simulink model "sim_tase_2025_att_ctrl"  (R2020a)
settings: Solver=ode4  StartTime=0.0  StopTime=30.0  FixedStep=0.01  RelTol=1e-3
values from neighbouring files (symbols this model uses):
  alfa_i_init = zeros(3, NF)    [init_tase_2025_att_ctrl.m]
  beta_ij_init = zeros(3, NF)    [init_tase_2025_att_ctrl.m]
  c1 = 2.5    [init_tase_2025_att_ctrl.m]
  c1_diff_sigma_bar_w = diag([12; 12; 12])    [init_tase_2025_att_ctrl.m]
  c1_diff_ui = diag([25; 30; 20])    [init_tase_2025_att_ctrl.m]
  c2 = 2.0    (= 2)    [init_tase_2025_att_ctrl.m]
  c2_diff_sigma_bar_w = diag([12; 12; 12])    [init_tase_2025_att_ctrl.m]
  c2_diff_ui = diag([50; 50; 10])    [init_tase_2025_att_ctrl.m]
  c3_diff_sigma_bar_w = diag([15; 15; 15])    [init_tase_2025_att_ctrl.m]
  c3_diff_ui = diag([15; 15; 10])    [init_tase_2025_att_ctrl.m]
  dw_aa_t = 0.2 * ones(3, 5) + ( 1.0 - 0.2 ) * rand(3, 5)    [init_tase_2025_att_ctrl.m]
  dw_ff_t = [ 0.4 * ones(1, 5) + ( 1.0 - 0.4 ) * rand(1, 5);                      0.4 * ones(1, 5) + ( 1.0 - 0.4 ) * rand(1, 5);                      0.2 * ones(1, 5) + ( 0.6 - 0.2 ) * rand(1, 5) ]    [init_tase_2025_att_ctrl.m]
  dw_phi_t = ( - pi / 2 ) * ones(3, 5) + ( pi / 2 - ( - pi / 2 ) ) * rand(3, 5)    [init_tase_2025_att_ctrl.m]
  dwci_init = zeros(3,5)    [init_tase_2025_att_ctrl.m]
  err_wi_init = zeros(3, NF)    [init_tase_2025_att_ctrl.m]
  eta_1_ij_init = zeros(3, NF)    [init_tase_2025_att_ctrl.m]
  eta_2_ij_init = zeros(3, NF)    [init_tase_2025_att_ctrl.m]
  h1w = diag([20.0; 20.0; 20.0])    [init_tase_2025_att_ctrl.m]
  h2w = diag([30.0; 35.0; 35.0])    [init_tase_2025_att_ctrl.m]
  h3w = diag([30.0; 25.0; 30.0])    [init_tase_2025_att_ctrl.m]
  Ji = zeros(3,3,NF)    [init_tase_2025_att_ctrl.m]
  k_1_ij_hat_init = zeros(3, NF)    [init_tase_2025_att_ctrl.m]
  k_1_ij_init = zeros(3, NF)    [init_tase_2025_att_ctrl.m]
  k_1_ij_lower = zeros(3, NF)    [init_tase_2025_att_ctrl.m]
  k_1_ij_upper = zeros(3, NF)    [init_tase_2025_att_ctrl.m]
  k_2_ij_init = zeros(3, NF)    [init_tase_2025_att_ctrl.m]
  k_2_ij_lower = zeros(3, NF)    [init_tase_2025_att_ctrl.m]
  k_2_ij_upper = zeros(3, NF)    [init_tase_2025_att_ctrl.m]
  Lamd_diff_sigma_bar_w = 0.8    [init_tase_2025_att_ctrl.m]
  Lamd_diff_ui = 0.8    [init_tase_2025_att_ctrl.m]
  mu1 = 0.2    [init_tase_2025_att_ctrl.m]
  mu2 = 0.2    [init_tase_2025_att_ctrl.m]
  mu_d_w = 100    [init_tase_2025_att_ctrl.m]
  phi_ij_init = ones(3, NF)    [init_tase_2025_att_ctrl.m]
  pos0 = zeros(3, 1)    [init_tase_2025_att_ctrl.m]
  PZ0 = P0(3)    [init_tase_2025_att_ctrl.m]
  PZ1 = 10    [init_tase_2025_att_ctrl.m]
  q_ij_hat_init = zeros(3, NF)    [init_tase_2025_att_ctrl.m]
  Qci_init = repmat([1;0;0;0],1,NF)    [init_tase_2025_att_ctrl.m]
  R0 = 4    [init_tase_2025_att_ctrl.m]
  R1 = 8    [init_tase_2025_att_ctrl.m]
  Rci_init = zeros(3,3,NF)    [init_tase_2025_att_ctrl.m]
  Ri_init = zeros(3,3,NF)    [init_tase_2025_att_ctrl.m]
  Rx2 = 10    [init_tase_2025_att_ctrl.m]
  Ry2 = 6    [init_tase_2025_att_ctrl.m]
  Rz2 = 4    [init_tase_2025_att_ctrl.m]
  T0 = 0    [init_tase_2025_att_ctrl.m]
  T1 = tseq1    (= 10)    [init_tase_2025_att_ctrl.m]
  T2 = tseq1 + tseq12 + tseq2    (= 30)    [init_tase_2025_att_ctrl.m]
  T_ij = repmat([60.0; 60.0; 60.0], 1, NF)    [init_tase_2025_att_ctrl.m]
  ui_init = zeros(3,NF)    [init_tase_2025_att_ctrl.m]
  vel0 = zeros(3, 1)    [init_tase_2025_att_ctrl.m]
  wci_init = zeros(3,5)    [init_tase_2025_att_ctrl.m]
  zeta_diff_sigma_bar_w = 0.3    [init_tase_2025_att_ctrl.m]
  zeta_diff_ui = 0.05    [init_tase_2025_att_ctrl.m]
undefined symbols (not defined in the file or in its folder): cal_frac_squ, p_alfaw1, p_alfaw2, q_alfaw1, q_alfaw2, Qei_init, Qi_init, Rei_init, V_Phi_Rei_init, wei_init, wi_init
(part 4 of 5)

== matlab function sim_tase_2025_att_ctrl/combine wei Qei Rei ==
  data: wei_1 input; wei_vec output; wei_2 input; wei_3 input; wei_4 input; wei_5 input; Qei_1 input; Qei_2 input; Qei_3 input; Qei_4 input; Qei_5 input; Rei_1 input; Rei_2 input; Rei_3 input; Rei_4 input; Rei_5 input; Qei_vec output; Rei_vec output
function [wei_vec, Qei_vec, Rei_vec] = fcn(wei_1, wei_2, wei_3, wei_4, wei_5, ...
                                                                            Qei_1, Qei_2, Qei_3, Qei_4, Qei_5, ...
                                                                            Rei_1, Rei_2, Rei_3, Rei_4, Rei_5)
%%%% 合并姿态角速率误差/四元数误差/姿态旋转矩阵误差
wei_vec = zeros(3,5);
wei_vec(:,1) = wei_1(:);
wei_vec(:,2) = wei_2(:);
wei_vec(:,3) = wei_3(:);
wei_vec(:,4) = wei_4(:);
wei_vec(:,5) = wei_5(:);

Qei_vec = zeros(4,5);
Qei_vec(:,1) = Qei_1(:);
Qei_vec(:,2) = Qei_2(:);
Qei_vec(:,3) = Qei_3(:);
Qei_vec(:,4) = Qei_4(:);
Qei_vec(:,5) = Qei_5(:);

Rei_vec = zeros(3,3,5);
Rei_vec(:,:,1) = Rei_1;
Rei_vec(:,:,2) = Rei_2;
Rei_vec(:,:,3) = Rei_3;
Rei_vec(:,:,4) = Rei_4;
Rei_vec(:,:,5) = Rei_5;

== matlab function sim_tase_2025_att_ctrl/cal Ri agent 1 ==
  data: Ri_1 output; Qi_vec input
function Ri_1 = fcn(Qi_vec)
%%%% 使用罗德里格公式由四元数Qi求解Ri
iiuav = 1;
thetai_tmp = Qi_vec(1,iiuav);
qi_tmp = Qi_vec(2:4,iiuav);
Ri_1 = ((thetai_tmp^2) - (qi_tmp')*qi_tmp) * eye(3,3) ...
            + 2 * qi_tmp * (qi_tmp') ...
            - 2 * thetai_tmp * cal_askew_mat(qi_tmp);

end

== matlab function sim_tase_2025_att_ctrl/cal Ri agent 2 ==
  data: Ri_2 output; Qi_vec input
function Ri_2 = fcn(Qi_vec)
%%%% 使用罗德里格公式由四元数Qi求解Ri
iiuav = 2;
thetai_tmp = Qi_vec(1,iiuav);
qi_tmp = Qi_vec(2:4,iiuav);
Ri_2 = ((thetai_tmp^2) - (qi_tmp')*qi_tmp) * eye(3,3) ...
            + 2 * qi_tmp * (qi_tmp') ...
            - 2 * thetai_tmp * cal_askew_mat(qi_tmp);

end

== matlab function sim_tase_2025_att_ctrl/combine phi_ij ==
  data: phi_ij_1 input; phi_ij_vec output; phi_ij_2 input; phi_ij_3 input; phi_ij_4 input; phi_ij_5 input
function phi_ij_vec = fcn(phi_ij_1, phi_ij_2, phi_ij_3, phi_ij_4, phi_ij_5)
%%%% 合并性能调节函数
phi_ij_vec = [phi_ij_1(:), phi_ij_2(:), phi_ij_3(:), phi_ij_4(:), phi_ij_5(:)];

== matlab function sim_tase_2025_att_ctrl/cal Ri agent 3 ==
  data: Ri_3 output; Qi_vec input
function Ri_3 = fcn(Qi_vec)
%%%% 使用罗德里格公式由四元数Qi求解Ri
iiuav = 3;
thetai_tmp = Qi_vec(1,iiuav);
qi_tmp = Qi_vec(2:4,iiuav);
Ri_3 = ((thetai_tmp^2) - (qi_tmp')*qi_tmp) * eye(3,3) ...
            + 2 * qi_tmp * (qi_tmp') ...
            - 2 * thetai_tmp * cal_askew_mat(qi_tmp);

end

== matlab function sim_tase_2025_att_ctrl/cal Ri agent 4 ==
  data: Ri_4 output; Qi_vec input
function Ri_4 = fcn(Qi_vec)
%%%% 使用罗德里格公式由四元数Qi求解Ri
iiuav = 4;
thetai_tmp = Qi_vec(1,iiuav);
qi_tmp = Qi_vec(2:4,iiuav);
Ri_4 = ((thetai_tmp^2) - (qi_tmp')*qi_tmp) * eye(3,3) ...
            + 2 * qi_tmp * (qi_tmp') ...
            - 2 * thetai_tmp * cal_askew_mat(qi_tmp);

end

== matlab function sim_tase_2025_att_ctrl/cal Ri agent 5 ==
  data: Ri_5 output; Qi_vec input
function Ri_5 = fcn(Qi_vec)
%%%% 使用罗德里格公式由四元数Qi求解Ri
iiuav = 5;
thetai_tmp = Qi_vec(1,iiuav);
qi_tmp = Qi_vec(2:4,iiuav);
Ri_5 = ((thetai_tmp^2) - (qi_tmp')*qi_tmp) * eye(3,3) ...
            + 2 * qi_tmp * (qi_tmp') ...
            - 2 * thetai_tmp * cal_askew_mat(qi_tmp);

end

== matlab function sim_tase_2025_att_ctrl/cal Qci agent 1 ==
  data: Qi_vec input; Qci_1 output; Qei_vec input
function Qci_1 = fcn(Qi_vec, Qei_vec)
%%%% 更新期望指令四元数
iiuav = 1;

sigma1 = Qi_vec(1,iiuav);
q1 = Qi_vec(2:4,iiuav);
sigma2 = Qei_vec(1,iiuav);
q2 = -Qei_vec(2:4,iiuav);

sigma = sigma1*sigma2 - (q1')*q2;
q = sigma1*q2 + sigma2*q1 + cal_askew_mat(q1)*q2;
Qci_1 = [sigma; q];

end

== matlab function sim_tase_2025_att_ctrl/cal Rci agent 1 ==
  data: Rci_1 output; Qci input
function Rci_1 = fcn(Qci)
%%%% 使用罗德里格公式由四元数Qci求解Rci
thetaci_tmp = Qci(1,1);
qci_tmp = Qci(2:4,1);
Rci_1 = ((thetaci_tmp^2) - (qci_tmp')*qci_tmp) * eye(3,3) ...
                + 2 * qci_tmp * (qci_tmp') ...
                - 2 * thetaci_tmp * cal_askew_mat(qci_tmp);

end

== matlab function sim_tase_2025_att_ctrl/cal Qci agent 2 ==
  data: Qi_vec input; Qci_2 output; Qei_vec input
function Qci_2 = fcn(Qi_vec, Qei_vec)
%%%% 更新期望指令四元数
iiuav = 2;
sigma1 = Qi_vec(1,iiuav);
q1 = Qi_vec(2:4,iiuav);
sigma2 = Qei_vec(1,iiuav);
q2 = -Qei_vec(2:4,iiuav);

sigma = sigma1*sigma2 - (q1')*q2;
q = sigma1*q2 + sigma2*q1 + cal_askew_mat(q1)*q2;
Qci_2 = [sigma; q];

end

== matlab function sim_tase_2025_att_ctrl/cal Rci agent 2 ==
  data: Rci_2 output; Qci input
function Rci_2 = fcn(Qci)
%%%% 使用罗德里格公式由四元数Qci求解Rci

thetaci_tmp = Qci(1,1);
qci_tmp = Qci(2:4,1);
Rci_2 = ((thetaci_tmp^2) - (qci_tmp')*qci_tmp) * eye(3,3) ...
                + 2 * qci_tmp * (qci_tmp') ...
                - 2 * thetaci_tmp * cal_askew_mat(qci_tmp);

end

== matlab function sim_tase_2025_att_ctrl/cal Qci agent 3 ==
  data: Qi_vec input; Qci_3 output; Qei_vec input
function Qci_3 = fcn(Qi_vec, Qei_vec)
%%%% 更新期望指令四元数
iiuav = 3;
sigma1 = Qi_vec(1,iiuav);
q1 = Qi_vec(2:4,iiuav);
sigma2 = Qei_vec(1,iiuav);
q2 = -Qei_vec(2:4,iiuav);

sigma = sigma1*sigma2 - (q1')*q2;
q = sigma1*q2 + sigma2*q1 + cal_askew_mat(q1)*q2;
Qci_3 = [sigma; q];

end

== matlab function sim_tase_2025_att_ctrl/cal Rci agent 3 ==
  data: Rci_3 output; Qci input
function Rci_3 = fcn(Qci)
%%%% 使用罗德里格公式由四元数Qci求解Rci
thetaci_tmp = Qci(1,1);
qci_tmp = Qci(2:4,1);
Rci_3 = ((thetaci_tmp^2) - (qci_tmp')*qci_tmp) * eye(3,3) ...
                + 2 * qci_tmp * (qci_tmp') ...
                - 2 * thetaci_tmp * cal_askew_mat(qci_tmp);

end

== matlab function sim_tase_2025_att_ctrl/cal Qci agent 4 ==
  data: Qi_vec input; Qci_4 output; Qei_vec input
function Qci_4 = fcn(Qi_vec, Qei_vec)
%%%% 更新期望指令四元数
iiuav = 4;
sigma1 = Qi_vec(1,iiuav);
q1 = Qi_vec(2:4,iiuav);
sigma2 = Qei_vec(1,iiuav);
q2 = -Qei_vec(2:4,iiuav);

sigma = sigma1*sigma2 - (q1')*q2;
q = sigma1*q2 + sigma2*q1 + cal_askew_mat(q1)*q2;
Qci_4 = [sigma; q];

end

== matlab function sim_tase_2025_att_ctrl/cal Rci agent 4 ==
  data: Rci_4 output; Qci input
function Rci_4 = fcn(Qci)
%%%% 使用罗德里格公式由四元数Qci求解Rci
thetaci_tmp = Qci(1,1);
qci_tmp = Qci(2:4,1);
Rci_4 = ((thetaci_tmp^2) - (qci_tmp')*qci_tmp) * eye(3,3) ...
                + 2 * qci_tmp * (qci_tmp') ...
                - 2 * thetaci_tmp * cal_askew_mat(qci_tmp);

end

== matlab function sim_tase_2025_att_ctrl/cal Qci agent 5 ==
  data: Qi_vec input; Qci_5 output; Qei_vec input
function Qci_5 = fcn(Qi_vec, Qei_vec)
%%%% 更新期望指令四元数
iiuav = 5;
sigma1 = Qi_vec(1,iiuav);
q1 = Qi_vec(2:4,iiuav);
sigma2 = Qei_vec(1,iiuav);
q2 = -Qei_vec(2:4,iiuav);

sigma = sigma1*sigma2 - (q1')*q2;
q = sigma1*q2 + sigma2*q1 + cal_askew_mat(q1)*q2;
Qci_5 = [sigma; q];

end

== matlab function sim_tase_2025_att_ctrl/cal Rci agent 5 ==
  data: Rci_5 output; Qci_vec input
function Rci_5 = fcn(Qci_vec)
%%%% 使用罗德里格公式由四元数Qci求解Rci
thetaci_tmp = Qci_vec(1,1);
qci_tmp = Qci_vec(2:4,1);
Rci_5 = ((thetaci_tmp^2) - (qci_tmp')*qci_tmp) * eye(3,3) ...
                + 2 * qci_tmp * (qci_tmp') ...
                - 2 * thetaci_tmp * cal_askew_mat(qci_tmp);

end

== matlab function sim_tase_2025_att_ctrl/combine Qci Rci ==
  data: Qci_1 input; Qci_vec output; Qci_2 input; Qci_3 input; Qci_4 input; Qci_5 input; Rci_1 input; Rci_2 input; Rci_3 input; Rci_4 input; Rci_5 input; Rci_vec output
function [Qci_vec, Rci_vec] = fcn(Qci_1, Qci_2, Qci_3, Qci_4, Qci_5, ...
                                                            Rci_1, Rci_2, Rci_3, Rci_4, Rci_5)
%%%% 合并四元数和姿态旋转矩阵
Qci_vec = zeros(4,5);
Qci_vec(:,1) = Qci_1(:);
Qci_vec(:,2) = Qci_2(:);
Qci_vec(:,3) = Qci_3(:);
Qci_vec(:,4) = Qci_4(:);
Qci_vec(:,5) = Qci_5(:);

Rci_vec = zeros(3,3,5);
Rci_vec(:,:,1) = Rci_1;
Rci_vec(:,:,2) = Rci_2;
Rci_vec(:,:,3) = Rci_3;
Rci_vec(:,:,4) = Rci_4;
Rci_vec(:,:,5) = Rci_5;

== matlab function sim_tase_2025_att_ctrl/cal k_1_ij agent 1 ==
  data: mu1 input; k_1_ij_lower input; k_1_ij_node_1 output; k_1_ij_upper input; phi_ij_vec input; tsim input
function k_1_ij_node_1 = fcn(mu1, k_1_ij_lower, k_1_ij_upper, phi_ij_vec, tsim)
%%%% 计算预设性能函数
iiuav = 1;
k_1_ij_node_1 = zeros(3,1);
for jj = 1:3
    k_1_ij_node_1(jj) = k_1_ij_lower(jj, iiuav) + ( k_1_ij_upper(jj, iiuav) - k_1_ij_lower(jj, iiuav) ) * phi_ij_vec(jj, iiuav);
%     k_1_ij_node_1(jj) = k_1_ij_lower(jj, iiuav) + ( k_1_ij_upper(jj, iiuav) - k_1_ij_lower(jj, iiuav) ) * phi_ij_vec(jj, iiuav) * exp( - mu1 * tsim );
%     k_1_ij_node_1(jj) = k_1_ij_lower(jj, iiuav) + ( k_1_ij_upper(jj, iiuav) - k_1_ij_lower(jj, iiuav) ) * exp( - mu1 * tsim );
end

== matlab function sim_tase_2025_att_ctrl/depart eta_1_ij 5 ==
  data: y output; x input
function y = fcn(x)
y = x(:,5);

end

== matlab function sim_tase_2025_att_ctrl/depart eta_1_ij 1 ==
  data: y output; x input
function y = fcn(x)
y = x(:,1);

end

== matlab function sim_tase_2025_att_ctrl/depart eta_1_ij 2 ==
  data: y output; x input
function y = fcn(x)
y = x(:,2);

end

== matlab function sim_tase_2025_att_ctrl/depart eta_1_ij 3 ==
  data: y output; x input
function y = fcn(x)
y = x(:,3);

end

== matlab function sim_tase_2025_att_ctrl/depart eta_1_ij 4 ==
  data: y output; x input
function y = fcn(x)
y = x(:,4);

end

== matlab function sim_tase_2025_att_ctrl/depart eta_2_ij 5 ==
  data: y output; x input
function y = fcn(x)
y = x(:,5);

end

== matlab function sim_tase_2025_att_ctrl/depart eta_2_ij 1 ==
  data: y output; x input
function y = fcn(x)
y = x(:,1);

end

== matlab function sim_tase_2025_att_ctrl/depart eta_2_ij 2 ==
  data: y output; x input
function y = fcn(x)
y = x(:,2);

end

== matlab function sim_tase_2025_att_ctrl/depart eta_2_ij 3 ==
  data: y output; x input
function y = fcn(x)
y = x(:,3);

end

== matlab function sim_tase_2025_att_ctrl/depart eta_2_ij 4 ==
  data: y output; x input
function y = fcn(x)
y = x(:,4);

end

== matlab function sim_tase_2025_att_ctrl/cal V_Phi_Rei agent 1 ==
  data: Rei_vec input; V_Phi_Rei_1 output
function V_Phi_Rei_1 = fcn(Rei_vec)
%%%% 更新姿态旋转指数坐标
iiuav = 1;
phiei = 0.5 * ( trace( Rei_vec(:,:,iiuav) ) - 1 );
V_Phi_Rei_1 = ( phiei / ( 2 * sin( phiei ) ) ) * ...
                            cal_back_askew_mat( Rei_vec(:,:,iiuav) - ( Rei_vec(:,:,iiuav)' ) );
end

== matlab function sim_tase_2025_att_ctrl/cal V_Phi_Rei agent 2 ==
  data: Rei_vec input; V_Phi_Rei_2 output
function V_Phi_Rei_2 = fcn(Rei_vec)
%%%% 更新姿态旋转指数坐标
iiuav = 2;
phiei = 0.5 * ( trace( Rei_vec(:,:,iiuav) ) - 1 );
V_Phi_Rei_2 = ( phiei / ( 2 * sin( phiei ) ) ) * ...
                            cal_back_askew_mat( Rei_vec(:,:,iiuav) - ( Rei_vec(:,:,iiuav)' ) );
end

== matlab function sim_tase_2025_att_ctrl/cal V_Phi_Rei agent 3 ==
  data: Rei_vec input; V_Phi_Rei_3 output
function V_Phi_Rei_3 = fcn(Rei_vec)
%%%% 更新姿态旋转指数坐标
iiuav = 3;
phiei = 0.5 * ( trace( Rei_vec(:,:,iiuav) ) - 1 );
V_Phi_Rei_3 = ( phiei / ( 2 * sin( phiei ) ) ) * ...
                            cal_back_askew_mat( Rei_vec(:,:,iiuav) - ( Rei_vec(:,:,iiuav)' ) );
end

== matlab function sim_tase_2025_att_ctrl/cal V_Phi_Rei agent 4 ==
  data: Rei_vec input; V_Phi_Rei_4 output
function V_Phi_Rei_4 = fcn(Rei_vec)
%%%% 更新姿态旋转指数坐标
iiuav = 4;
phiei = 0.5 * ( trace( Rei_vec(:,:,iiuav) ) - 1 );
V_Phi_Rei_4 = ( phiei / ( 2 * sin( phiei ) ) ) * ...
                            cal_back_askew_mat( Rei_vec(:,:,iiuav) - ( Rei_vec(:,:,iiuav)' ) );
end

== matlab function sim_tase_2025_att_ctrl/cal V_Phi_Rei agent 5 ==
  data: Rei_vec input; V_Phi_Rei_5 output
function V_Phi_Rei_5 = fcn(Rei_vec)
%%%% 更新姿态旋转指数坐标
iiuav = 5;
phiei = 0.5 * ( trace( Rei_vec(:,:,iiuav) ) - 1 );
V_Phi_Rei_5 = ( phiei / ( 2 * sin( phiei ) ) ) * ...
                            cal_back_askew_mat( Rei_vec(:,:,iiuav) - ( Rei_vec(:,:,iiuav)' ) );
end

== matlab function sim_tase_2025_att_ctrl/cal k_1_ij agent 2 ==
  data: mu1 input; k_1_ij_lower input; k_1_ij_node_2 output; k_1_ij_upper input; phi_ij_vec input; tsim input
function k_1_ij_node_2 = fcn(mu1, k_1_ij_lower, k_1_ij_upper, phi_ij_vec, tsim)
%%%% 计算预设性能函数
iiuav = 2;
k_1_ij_node_2 = zeros(3,1);
for jj = 1:3
    k_1_ij_node_2(jj) = k_1_ij_lower(jj, iiuav) + ( k_1_ij_upper(jj, iiuav) - k_1_ij_lower(jj, iiuav) ) * phi_ij_vec(jj, iiuav);
%     k_1_ij_node_2(jj) = k_1_ij_lower(jj, iiuav) + ( k_1_ij_upper(jj, iiuav) - k_1_ij_lower(jj, iiuav) ) * phi_ij_vec(jj, iiuav) * exp( - mu1 * tsim );
%     k_1_ij_node_2(jj) = k_1_ij_lower(jj, iiuav) + ( k_1_ij_upper(jj, iiuav) - k_1_ij_lower(jj, iiuav) ) * exp( - mu1 * tsim );
end

== matlab function sim_tase_2025_att_ctrl/cal differentiator d_sigma_bar_w_hat agent 3/choose sigma_bar_w ==
  data: x input; y output
function y = fcn(x)
iiuav = 3;
y = x(:,iiuav);

== matlab function sim_tase_2025_att_ctrl/cal differentiator d_sigma_bar_w_hat agent 3/trans to column20 ==
  data: x input; y output
function y = fcn(x)
y = x(:);

== matlab function sim_tase_2025_att_ctrl/cal differentiator d_sigma_bar_w_hat agent 3/trans to column21 ==
  data: x input; y output
function y = fcn(x)
y = x(:);

== matlab function sim_tase_2025_att_ctrl/cal differentiator d_sigma_bar_w_hat agent 3/trans to column22 ==
  data: x input; y output
function y = fcn(x)
y = x(:);

== matlab function sim_tase_2025_att_ctrl/cal differentiator d_sigma_bar_w_hat agent 3/trans to column23 ==
  data: x input; y output
function y = fcn(x)
y = x(:);

== matlab function sim_tase_2025_att_ctrl/combine Qci Rci1 ==
  data: V_Phi_Rei_1 input; V_Phi_Rei_vec output; V_Phi_Rei_2 input; V_Phi_Rei_3 input; V_Phi_Rei_4 input; V_Phi_Rei_5 input
function V_Phi_Rei_vec = fcn(V_Phi_Rei_1, V_Phi_Rei_2, V_Phi_Rei_3, V_Phi_Rei_4, V_Phi_Rei_5)
%%%% 合并LogSO3空间的辅助姿态误差向量
V_Phi_Rei_vec = [V_Phi_Rei_1(:), V_Phi_Rei_2(:), V_Phi_Rei_3(:), V_Phi_Rei_4(:), V_Phi_Rei_5(:)];

== matlab function sim_tase_2025_att_ctrl/depart Qe1 ==
  data: y output; x input
function y = fcn(x)
y = x(:,1);

end

== matlab function sim_tase_2025_att_ctrl/depart Qe2 ==
  data: y output; x input
function y = fcn(x)
y = x(:,2);

end

== matlab function sim_tase_2025_att_ctrl/depart Qe3 ==
  data: y output; x input
function y = fcn(x)
y = x(:,3);

end

== matlab function sim_tase_2025_att_ctrl/depart Qe4 ==
  data: y output; x input
function y = fcn(x)
y = x(:,4);

end

== matlab function sim_tase_2025_att_ctrl/depart Qe5 ==
  data: y output; x input
function y = fcn(x)
y = x(:,5);

end

== matlab function sim_tase_2025_att_ctrl/depart we1 ==
  data: y output; x input
function y = fcn(x)
y = x(:,1);

end

== matlab function sim_tase_2025_att_ctrl/depart we2 ==
  data: y output; x input
function y = fcn(x)
y = x(:,2);

end

== matlab function sim_tase_2025_att_ctrl/depart we3 ==
  data: y output; x input
function y = fcn(x)
y = x(:,3);

end

== matlab function sim_tase_2025_att_ctrl/depart we4 ==
  data: y output; x input
function y = fcn(x)
y = x(:,4);

end

== matlab function sim_tase_2025_att_ctrl/cal k_1_ij agent 3 ==
  data: mu1 input; k_1_ij_lower input; k_1_ij_node_3 output; k_1_ij_upper input; phi_ij_vec input; tsim input
function k_1_ij_node_3 = fcn(mu1, k_1_ij_lower, k_1_ij_upper, phi_ij_vec, tsim)
%%%% 计算预设性能函数
iiuav = 3;
k_1_ij_node_3 = zeros(3,1);
for jj = 1:3
    k_1_ij_node_3(jj) = k_1_ij_lower(jj, iiuav) + ( k_1_ij_upper(jj, iiuav) - k_1_ij_lower(jj, iiuav) ) * phi_ij_vec(jj, iiuav);
%     k_1_ij_node_3(jj) = k_1_ij_lower(jj, iiuav) + ( k_1_ij_upper(jj, iiuav) - k_1_ij_lower(jj, iiuav) ) * phi_ij_vec(jj, iiuav) * exp( - mu1 * tsim );
%     k_1_ij_node_3(jj) = k_1_ij_lower(jj, iiuav) + ( k_1_ij_upper(jj, iiuav) - k_1_ij_lower(jj, iiuav) ) * exp( - mu1 * tsim );
end

== matlab function sim_tase_2025_att_ctrl/depart we5 ==
  data: y output; x input
function y = fcn(x)
y = x(:,5);

end

== matlab function sim_tase_2025_att_ctrl/depart V_Phi_Re5 ==
  data: y output; x input
function y = fcn(x)
y = x(:,5);

end

== matlab function sim_tase_2025_att_ctrl/depart V_Phi_Re1 ==
  data: y output; x input
function y = fcn(x)
y = x(:,1);

end

== matlab function sim_tase_2025_att_ctrl/depart V_Phi_Re2 ==
  data: y output; x input
function y = fcn(x)
y = x(:,2);

end

== matlab function sim_tase_2025_att_ctrl/depart V_Phi_Re3 ==
  data: y output; x input
function y = fcn(x)
y = x(:,3);

end

== matlab function sim_tase_2025_att_ctrl/depart V_Phi_Re4 ==
  data: y output; x input
function y = fcn(x)
y = x(:,4);

end

== matlab function sim_tase_2025_att_ctrl/cal differentiator d_sigma_bar_w_hat agent 3/trans to column24 ==
  data: x input; y output
function y = fcn(x)
y = x(:);

== matlab function sim_tase_2025_att_ctrl/cal differentiator d_sigma_bar_w_hat agent 3/trans to column25 ==
  data: x input; y output
function y = fcn(x)
y = x(:);

== matlab function sim_tase_2025_att_ctrl/cal differentiator d_sigma_bar_w_hat agent 4/cal differentiator ==
  data: c1 input; d_sigma_bar_v_hat output; d_dsigma_bar_v_hat output; d_d2sigma_bar_v_hat output; c2 input; c3 input; chi_t input; sigma_bar_v_sig_1 input; sigma_bar_v_sig_2 input; sigma_bar_v_sig_3 input; sigma_bar_v_sig_4 input; sigma_bar_v_sig_5 input; sigma_bar_v_sig_6 input; d_sigma_bar_v_hat input; d2_sigma_bar_v_hat input
function [d_sigma_bar_v_hat, d_dsigma_bar_v_hat, d_d2sigma_bar_v_hat] = fcn(c1, c2, c3, chi_t, sigma_bar_v_sig_1, sigma_bar_v_sig_2, sigma_bar_v_sig_3, ...
                                                                                                                                                sigma_bar_v_sig_4, sigma_bar_v_sig_5, sigma_bar_v_sig_6, d_sigma_bar_v_hat, d2_sigma_bar_v_hat)
d_d2sigma_bar_v_hat = -chi_t .* c1 * sigma_bar_v_sig_1(:) - (1 - chi_t) .* c1 * sigma_bar_v_sig_2(:);
d_dsigma_bar_v_hat = -chi_t .* c2 * sigma_bar_v_sig_3(:) - (1 - chi_t) .* c2 * sigma_bar_v_sig_4(:) + d2_sigma_bar_v_hat(:);
d_sigma_bar_v_hat = -chi_t .* c3 * sigma_bar_v_sig_5(:) - (1 - chi_t) .* c3 * sigma_bar_v_sig_6(:) + d_sigma_bar_v_hat(:);

== matlab function sim_tase_2025_att_ctrl/cal differentiator d_sigma_bar_w_hat agent 4/cal sig ==
  data: x input; z output; y input
function z = fcn(x, y)
z = x(:) .* sign(y(:));

== matlab function sim_tase_2025_att_ctrl/cal differentiator d_sigma_bar_w_hat agent 4/cal sig1 ==
  data: x input; z output; y input
function z = fcn(x, y)
z = x(:) .* sign(y(:));

== matlab function sim_tase_2025_att_ctrl/cal differentiator d_sigma_bar_w_hat agent 4/cal sig2 ==
  data: x input; z output; y input
function z = fcn(x, y)
z = x(:) .* sign(y(:));

== matlab function sim_tase_2025_att_ctrl/cal differentiator d_sigma_bar_w_hat agent 4/cal sig3 ==
  data: x input; z output; y input
function z = fcn(x, y)
z = x(:) .* sign(y(:));

== matlab function sim_tase_2025_att_ctrl/cal k_1_ij agent 4 ==
  data: mu1 input; k_1_ij_lower input; k_1_ij_node_4 output; k_1_ij_upper input; phi_ij_vec input; tsim input
function k_1_ij_node_4 = fcn(mu1, k_1_ij_lower, k_1_ij_upper, phi_ij_vec, tsim)
%%%% 计算预设性能函数
iiuav = 4;
k_1_ij_node_4 = zeros(3,1);
for jj = 1:3
    k_1_ij_node_4(jj) = k_1_ij_lower(jj, iiuav) + ( k_1_ij_upper(jj, iiuav) - k_1_ij_lower(jj, iiuav) ) * phi_ij_vec(jj, iiuav);
%     k_1_ij_node_4(jj) = k_1_ij_lower(jj, iiuav) + ( k_1_ij_upper(jj, iiuav) - k_1_ij_lower(jj, iiuav) ) * phi_ij_vec(jj, iiuav) * exp( - mu1 * tsim );
%     k_1_ij_node_4(jj) = k_1_ij_lower(jj, iiuav) + ( k_1_ij_upper(jj, iiuav) - k_1_ij_lower(jj, iiuav) ) * exp( - mu1 * tsim );
end

== matlab function sim_tase_2025_att_ctrl/cal differentiator d_sigma_bar_w_hat agent 4/cal sig4 ==
  data: x input; z output; y input
function z = fcn(x, y)
z = x(:) .* sign(y(:));

== matlab function sim_tase_2025_att_ctrl/cal differentiator d_sigma_bar_w_hat agent 4/cal sig5 ==
  data: x input; z output; y input
function z = fcn(x, y)
z = x(:) .* sign(y(:));

== matlab function sim_tase_2025_att_ctrl/cal differentiator d_sigma_bar_w_hat agent 4/choose sigma_bar_w ==
  data: x input; y output
function y = fcn(x)
iiuav = 4;
y = x(:,iiuav);

== matlab function sim_tase_2025_att_ctrl/cal differentiator d_sigma_bar_w_hat agent 4/trans to column20 ==
  data: x input; y output
function y = fcn(x)
y = x(:);

== matlab function sim_tase_2025_att_ctrl/cal differentiator d_sigma_bar_w_hat agent 4/trans to column21 ==
  data: x input; y output
function y = fcn(x)
y = x(:);

== matlab function sim_tase_2025_att_ctrl/cal differentiator d_sigma_bar_w_hat agent 4/trans to column22 ==
  data: x input; y output
function y = fcn(x)
y = x(:);

== matlab function sim_tase_2025_att_ctrl/cal differentiator d_sigma_bar_w_hat agent 4/trans to column23 ==
  data: x input; y output
function y = fcn(x)
y = x(:);

== matlab function sim_tase_2025_att_ctrl/cal differentiator d_sigma_bar_w_hat agent 4/trans to column24 ==
  data: x input; y output
function y = fcn(x)
y = x(:);

== matlab function sim_tase_2025_att_ctrl/cal differentiator d_sigma_bar_w_hat agent 4/trans to column25 ==
  data: x input; y output
function y = fcn(x)
y = x(:);

== matlab function sim_tase_2025_att_ctrl/cal differentiator d_sigma_bar_w_hat agent 5/cal differentiator ==
  data: c1 input; d_sigma_bar_v_hat output; d_dsigma_bar_v_hat output; d_d2sigma_bar_v_hat output; c2 input; c3 input; chi_t input; sigma_bar_v_sig_1 input; sigma_bar_v_sig_2 input; sigma_bar_v_sig_3 input; sigma_bar_v_sig_4 input; sigma_bar_v_sig_5 input; sigma_bar_v_sig_6 input; d_sigma_bar_v_hat input; d2_sigma_bar_v_hat input
function [d_sigma_bar_v_hat, d_dsigma_bar_v_hat, d_d2sigma_bar_v_hat] = fcn(c1, c2, c3, chi_t, sigma_bar_v_sig_1, sigma_bar_v_sig_2, sigma_bar_v_sig_3, ...
                                                                                                                                                sigma_bar_v_sig_4, sigma_bar_v_sig_5, sigma_bar_v_sig_6, d_sigma_bar_v_hat, d2_sigma_bar_v_hat)
d_d2sigma_bar_v_hat = -chi_t .* c1 * sigma_bar_v_sig_1(:) - (1 - chi_t) .* c1 * sigma_bar_v_sig_2(:);
d_dsigma_bar_v_hat = -chi_t .* c2 * sigma_bar_v_sig_3(:) - (1 - chi_t) .* c2 * sigma_bar_v_sig_4(:) + d2_sigma_bar_v_hat(:);
d_sigma_bar_v_hat = -chi_t .* c3 * sigma_bar_v_sig_5(:) - (1 - chi_t) .* c3 * sigma_bar_v_sig_6(:) + d_sigma_bar_v_hat(:);

== matlab function sim_tase_2025_att_ctrl/cal differentiator d_sigma_bar_w_hat agent 5/cal sig ==
  data: x input; z output; y input
function z = fcn(x, y)
z = x(:) .* sign(y(:));

== matlab function sim_tase_2025_att_ctrl/cal differentiator d_sigma_bar_w_hat agent 5/cal sig1 ==
  data: x input; z output; y input
function z = fcn(x, y)
z = x(:) .* sign(y(:));

== matlab function sim_tase_2025_att_ctrl/cal differentiator d_sigma_bar_w_hat agent 5/cal sig2 ==
  data: x input; z output; y input
function z = fcn(x, y)
z = x(:) .* sign(y(:));

== matlab function sim_tase_2025_att_ctrl/cal differentiator d_sigma_bar_w_hat agent 5/cal sig3 ==
  data: x input; z output; y input
function z = fcn(x, y)
z = x(:) .* sign(y(:));

== matlab function sim_tase_2025_att_ctrl/cal k_1_ij agent 5 ==
  data: mu1 input; k_1_ij_lower input; k_1_ij_node_5 output; k_1_ij_upper input; phi_ij_vec input; tsim input
function k_1_ij_node_5 = fcn(mu1, k_1_ij_lower, k_1_ij_upper, phi_ij_vec, tsim)
%%%% 计算预设性能函数
iiuav = 5;
k_1_ij_node_5 = zeros(3,1);
for jj = 1:3
    k_1_ij_node_5(jj) = k_1_ij_lower(jj, iiuav) + ( k_1_ij_upper(jj, iiuav) - k_1_ij_lower(jj, iiuav) ) * phi_ij_vec(jj, iiuav);
%     k_1_ij_node_5(jj) = k_1_ij_lower(jj, iiuav) + ( k_1_ij_upper(jj, iiuav) - k_1_ij_lower(jj, iiuav) ) * phi_ij_vec(jj, iiuav) * exp( - mu1 * tsim );
%     k_1_ij_node_5(jj) = k_1_ij_lower(jj, iiuav) + ( k_1_ij_upper(jj, iiuav) - k_1_ij_lower(jj, iiuav) ) * exp( - mu1 * tsim );
end

== matlab function sim_tase_2025_att_ctrl/cal differentiator d_sigma_bar_w_hat agent 5/cal sig4 ==
  data: x input; z output; y input
function z = fcn(x, y)
z = x(:) .* sign(y(:));

== matlab function sim_tase_2025_att_ctrl/cal differentiator d_sigma_bar_w_hat agent 5/cal sig5 ==
  data: x input; z output; y input
function z = fcn(x, y)
z = x(:) .* sign(y(:));

== matlab function sim_tase_2025_att_ctrl/cal differentiator d_sigma_bar_w_hat agent 5/choose sigma_bar_w ==
  data: x input; y output
function y = fcn(x)
iiuav = 5;
y = x(:,iiuav);

== matlab function sim_tase_2025_att_ctrl/cal differentiator d_sigma_bar_w_hat agent 5/trans to column20 ==
  data: x input; y output
function y = fcn(x)
y = x(:);

== matlab function sim_tase_2025_att_ctrl/cal differentiator d_sigma_bar_w_hat agent 5/trans to column21 ==
  data: x input; y output
function y = fcn(x)
y = x(:);

== matlab function sim_tase_2025_att_ctrl/cal differentiator d_sigma_bar_w_hat agent 5/trans to column22 ==
  data: x input; y output
function y = fcn(x)
y = x(:);

== matlab function sim_tase_2025_att_ctrl/cal differentiator d_sigma_bar_w_hat agent 5/trans to column23 ==
  data: x input; y output
function y = fcn(x)
y = x(:);

== matlab function sim_tase_2025_att_ctrl/cal differentiator d_sigma_bar_w_hat agent 5/trans to column24 ==
  data: x input; y output
function y = fcn(x)
y = x(:);

== matlab function sim_tase_2025_att_ctrl/cal differentiator d_sigma_bar_w_hat agent 5/trans to column25 ==
  data: x input; y output
function y = fcn(x)
y = x(:);

== matlab function sim_tase_2025_att_ctrl/cal dw_hat agent 1 ==
  data: h3w input; Ji input; d_sigma_bar_w_vec input; sigma_bar_w_hat_vec input; dw_hat_1 output
function dw_hat_1 = fcn(h3w, Ji, d_sigma_bar_w_vec, sigma_bar_w_hat_vec)
%%%% 计算扰动观测值dw_hat
iiuav = 1;
dw_hat_1 = Ji(:,:,iiuav) * d_sigma_bar_w_vec(:,iiuav) + h3w * sigma_bar_w_hat_vec(:,iiuav);

== matlab function sim_tase_2025_att_ctrl/cal dw_hat agent 2 ==
  data: h3w input; Ji input; d_sigma_bar_w_vec input; sigma_bar_w_hat_vec input; dw_hat_2 output
function dw_hat_2 = fcn(h3w, Ji, d_sigma_bar_w_vec, sigma_bar_w_hat_vec)
%%%% 计算扰动观测值dw_hat
iiuav = 2;
dw_hat_2 = Ji(:,:,iiuav) * d_sigma_bar_w_vec(:,iiuav) + h3w * sigma_bar_w_hat_vec(:,iiuav);

== matlab function sim_tase_2025_att_ctrl/cal dw_hat agent 3 ==
  data: h3w input; Ji input; d_sigma_bar_w_vec input; sigma_bar_w_hat_vec input; dw_hat_3 output
function dw_hat_3 = fcn(h3w, Ji, d_sigma_bar_w_vec, sigma_bar_w_hat_vec)
%%%% 计算扰动观测值dw_hat
iiuav = 3;
dw_hat_3 = Ji(:,:,iiuav) * d_sigma_bar_w_vec(:,iiuav) + h3w * sigma_bar_w_hat_vec(:,iiuav);

== matlab function sim_tase_2025_att_ctrl/cal dw_hat agent 4 ==
  data: h3w input; Ji input; d_sigma_bar_w_vec input; sigma_bar_w_hat_vec input; dw_hat_4 output
function dw_hat_4 = fcn(h3w, Ji, d_sigma_bar_w_vec, sigma_bar_w_hat_vec)
%%%% 计算扰动观测值dw_hat
iiuav = 4;
dw_hat_4 = Ji(:,:,iiuav) * d_sigma_bar_w_vec(:,iiuav) + h3w * sigma_bar_w_hat_vec(:,iiuav);

== matlab function sim_tase_2025_att_ctrl/combine k_1_ij ==
  data: k_1_ij_node_1 input; k_1_ij_vec output; k_1_ij_node_2 input; k_1_ij_node_3 input; k_1_ij_node_4 input; k_1_ij_node_5 input
function k_1_ij_vec = fcn(k_1_ij_node_1, k_1_ij_node_2, k_1_ij_node_3, k_1_ij_node_4, k_1_ij_node_5)
%%%% 合并预设性能函数
k_1_ij_vec = [k_1_ij_node_1(:), k_1_ij_node_2(:), k_1_ij_node_3(:), k_1_ij_node_4(:), k_1_ij_node_5(:)];

== matlab function sim_tase_2025_att_ctrl/cal dw_hat agent 5 ==
  data: h3w input; Ji input; d_sigma_bar_w_vec input; sigma_bar_w_hat_vec input; dw_hat_5 output
function dw_hat_5 = fcn(h3w, Ji, d_sigma_bar_w_vec, sigma_bar_w_hat_vec)
%%%% 计算扰动观测值dw_hat
iiuav = 5;
dw_hat_5 = Ji(:,:,iiuav) * d_sigma_bar_w_vec(:,iiuav) + h3w * sigma_bar_w_hat_vec(:,iiuav);

== matlab function sim_tase_2025_att_ctrl/cal error dw_tilt ==
  data: dw_vec input; dw_hat_vec input; dw_tilt_vec output
function dw_tilt_vec = fcn(dw_vec, dw_hat_vec)
%%%% 计算扰动观测误差dw_tilt
dw_tilt_vec = zeros(3,5);
for iiuav = 1:5
    dw_tilt_vec(:,iiuav) = dw_vec(:,iiuav) - dw_hat_vec(:,iiuav);
end

== matlab function sim_tase_2025_att_ctrl/cal sigma_bar_w_hat agent 1 ==
  data: h1w input; h2w input; theta_sigma_bar_w_tilt_1_vec input; d_sigma_bar_w_hat_1 output; theta_sigma_bar_w_tilt_2_vec input; d_sigma_bar_w_vec input
function d_sigma_bar_w_hat_1 = fcn(h1w, h2w, theta_sigma_bar_w_tilt_1_vec, theta_sigma_bar_w_tilt_2_vec, d_sigma_bar_w_vec)
%%%% 计算扰动观测器中虚拟速度控制量观测值sigma_w_hat的微分方程
iiuav = 1;
d_sigma_bar_w_hat_1 = d_sigma_bar_w_vec(:,iiuav) + ...
                                            h1w * theta_sigma_bar_w_tilt_1_vec(:,iiuav) + ...
                                            h2w * theta_sigma_bar_w_tilt_2_vec(:,iiuav);

== matlab function sim_tase_2025_att_ctrl/cal sigma_bar_w_hat agent 2 ==
  data: h1w input; h2w input; theta_sigma_bar_w_tilt_1_vec input; d_sigma_bar_w_hat_2 output; theta_sigma_bar_w_tilt_2_vec input; d_sigma_bar_w_vec input
function d_sigma_bar_w_hat_2 = fcn(h1w, h2w, theta_sigma_bar_w_tilt_1_vec, theta_sigma_bar_w_tilt_2_vec, d_sigma_bar_w_vec)
%%%% 计算扰动观测器中虚拟速度控制量观测值sigma_v_hat的微分方程
iiuav = 2;
d_sigma_bar_w_hat_2 = d_sigma_bar_w_vec(:,iiuav) + ...
                                            h1w * theta_sigma_bar_w_tilt_1_vec(:,iiuav) + ...
                                            h2w * theta_sigma_bar_w_tilt_2_vec(:,iiuav);

== matlab function sim_tase_2025_att_ctrl/cal sigma_bar_w_hat agent 3 ==
  data: h1w input; h2w input; theta_sigma_bar_w_tilt_1_vec input; d_sigma_bar_w_hat_3 output; theta_sigma_bar_w_tilt_2_vec input; d_sigma_bar_w_vec input
function d_sigma_bar_w_hat_3 = fcn(h1w, h2w, theta_sigma_bar_w_tilt_1_vec, theta_sigma_bar_w_tilt_2_vec, d_sigma_bar_w_vec)
%%%% 计算扰动观测器中虚拟速度控制量观测值sigma_w_hat的微分方程
iiuav = 3;
d_sigma_bar_w_hat_3 = d_sigma_bar_w_vec(:,iiuav) + ...
                                            h1w * theta_sigma_bar_w_tilt_1_vec(:,iiuav) + ...
                                            h2w * theta_sigma_bar_w_tilt_2_vec(:,iiuav);

== matlab function sim_tase_2025_att_ctrl/cal sigma_bar_w_hat agent 4 ==
  data: h1w input; h2w input; theta_sigma_bar_w_tilt_1_vec input; d_sigma_bar_w_hat_4 output; theta_sigma_bar_w_tilt_2_vec input; d_sigma_bar_w_vec input
function d_sigma_bar_w_hat_4 = fcn(h1w, h2w, theta_sigma_bar_w_tilt_1_vec, theta_sigma_bar_w_tilt_2_vec, d_sigma_bar_w_vec)
%%%% 计算扰动观测器中虚拟速度控制量观测值sigma_w_hat的微分方程
iiuav = 4;
d_sigma_bar_w_hat_4 = d_sigma_bar_w_vec(:,iiuav) + ...
                                            h1w * theta_sigma_bar_w_tilt_1_vec(:,iiuav) + ...
                                            h2w * theta_sigma_bar_w_tilt_2_vec(:,iiuav);

== matlab function sim_tase_2025_att_ctrl/cal sigma_bar_w_hat agent 5 ==
  data: h1w input; h2w input; theta_sigma_bar_w_tilt_1_vec input; d_sigma_bar_w_hat_5 output; theta_sigma_bar_w_tilt_2_vec input; d_sigma_bar_w_vec input
function d_sigma_bar_w_hat_5 = fcn(h1w, h2w, theta_sigma_bar_w_tilt_1_vec, theta_sigma_bar_w_tilt_2_vec, d_sigma_bar_w_vec)
%%%% 计算扰动观测器中虚拟速度控制量观测值sigma_w_hat的微分方程
iiuav = 5;
d_sigma_bar_w_hat_5 = d_sigma_bar_w_vec(:,iiuav) + ...
                                            h1w * theta_sigma_bar_w_tilt_1_vec(:,iiuav) + ...
                                            h2w * theta_sigma_bar_w_tilt_2_vec(:,iiuav);

== matlab function sim_tase_2025_att_ctrl/cal sigma_w_bar ==
  data: sigma_bar_w_vec output; wi_vec input; sigma_w_vec input
function sigma_bar_w_vec = fcn(wi_vec, sigma_w_vec)
%%%% 计算姿态角速率跟踪误差
sigma_bar_w_vec = zeros(3,5);
for iiuav = 1:5
    sigma_bar_w_vec(:,iiuav) = wi_vec(:,iiuav) - sigma_w_vec(:,iiuav);
end

== matlab function sim_tase_2025_att_ctrl/cal theta_sigma_bar_w_tilt agent 1 ==
  data: alfa_theta_obs_w input; sigma_bar_w_tilt_squ_1_1 input; theta_sigma_bar_w_tilt_1_1 output; sigma_bar_w_tilt_squ_2_1 input; sigma_bar_w_tilt_vec input; theta_sigma_bar_w_tilt_2_1 output
function [theta_sigma_bar_w_tilt_1_1, theta_sigma_bar_w_tilt_2_1] = fcn(alfa_theta_obs_w, sigma_bar_w_tilt_squ_1_1, sigma_bar_w_tilt_squ_2_1, sigma_bar_w_tilt_vec)
%%%% 计算平滑递增函数
iiuav = 1;
theta_sigma_bar_w_tilt_1_1 = sigma_bar_w_tilt_squ_1_1(:) .* ( -1 + 2 ./ ( 1 + exp( -alfa_theta_obs_w .* sigma_bar_w_tilt_vec(:,iiuav) ) ) );
theta_sigma_bar_w_tilt_2_1 = sigma_bar_w_tilt_squ_2_1(:) .* ( -1 + 2 ./ ( 1 + exp( -alfa_theta_obs_w .* sigma_bar_w_tilt_vec(:,iiuav) ) ) );

== matlab function sim_tase_2025_att_ctrl/cal theta_sigma_bar_w_tilt agent 2 ==
  data: alfa_theta_obs_w input; sigma_bar_w_tilt_squ_1_2 input; theta_sigma_bar_w_tilt_1_2 output; sigma_bar_w_tilt_squ_2_2 input; sigma_bar_w_tilt_vec input; theta_sigma_bar_w_tilt_2_2 output
function [theta_sigma_bar_w_tilt_1_2, theta_sigma_bar_w_tilt_2_2] = fcn(alfa_theta_obs_w, sigma_bar_w_tilt_squ_1_2, sigma_bar_w_tilt_squ_2_2, sigma_bar_w_tilt_vec)
%%%% 计算平滑递增函数
iiuav = 2;
theta_sigma_bar_w_tilt_1_2 = sigma_bar_w_tilt_squ_1_2(:) .* ( -1 + 2 ./ ( 1 + exp( -alfa_theta_obs_w .* sigma_bar_w_tilt_vec(:,iiuav) ) ) );
theta_sigma_bar_w_tilt_2_2 = sigma_bar_w_tilt_squ_2_2(:) .* ( -1 + 2 ./ ( 1 + exp( -alfa_theta_obs_w .* sigma_bar_w_tilt_vec(:,iiuav) ) ) );

== matlab function sim_tase_2025_att_ctrl/cal theta_sigma_bar_w_tilt agent 3 ==
  data: alfa_theta_obs_w input; sigma_bar_w_tilt_squ_1_3 input; theta_sigma_bar_w_tilt_1_3 output; sigma_bar_w_tilt_squ_2_3 input; sigma_bar_w_tilt_vec input; theta_sigma_bar_w_tilt_2_3 output
function [theta_sigma_bar_w_tilt_1_3, theta_sigma_bar_w_tilt_2_3] = fcn(alfa_theta_obs_w, sigma_bar_w_tilt_squ_1_3, sigma_bar_w_tilt_squ_2_3, sigma_bar_w_tilt_vec)
%%%% 计算平滑递增函数
iiuav = 3;
theta_sigma_bar_w_tilt_1_3 = sigma_bar_w_tilt_squ_1_3(:) .* ( -1 + 2 ./ ( 1 + exp( -alfa_theta_obs_w .* sigma_bar_w_tilt_vec(:,iiuav) ) ) );
theta_sigma_bar_w_tilt_2_3 = sigma_bar_w_tilt_squ_2_3(:) .* ( -1 + 2 ./ ( 1 + exp( -alfa_theta_obs_w .* sigma_bar_w_tilt_vec(:,iiuav) ) ) );

== matlab function sim_tase_2025_att_ctrl/cal k_1_ij_hat agent 1 ==
  data: k_1_ij_lower input; k_1_ij_hat_node_1 output; k_1_ij_vec input
function k_1_ij_hat_node_1 = fcn(k_1_ij_lower, k_1_ij_vec)
%%%% 计算障碍函数
iiuav = 1;
k_1_ij_hat_node_1 = zeros(3,1);
for jj = 1:3
    k_1_ij_hat_node_1(jj) = (1/2) * ( k_1_ij_vec(jj,iiuav) + k_1_ij_lower(jj,iiuav) );
end

== matlab function sim_tase_2025_att_ctrl/cal theta_sigma_bar_w_tilt agent 4 ==
  data: alfa_theta_obs_w input; sigma_bar_w_tilt_squ_1_4 input; theta_sigma_bar_w_tilt_1_4 output; sigma_bar_w_tilt_squ_2_4 input; sigma_bar_w_tilt_vec input; theta_sigma_bar_w_tilt_2_4 output
function [theta_sigma_bar_w_tilt_1_4, theta_sigma_bar_w_tilt_2_4] = fcn(alfa_theta_obs_w, sigma_bar_w_tilt_squ_1_4, sigma_bar_w_tilt_squ_2_4, sigma_bar_w_tilt_vec)
%%%% 计算平滑递增函数
iiuav = 4;
theta_sigma_bar_w_tilt_1_4 = sigma_bar_w_tilt_squ_1_4(:) .* ( -1 + 2 ./ ( 1 + exp( -alfa_theta_obs_w .* sigma_bar_w_tilt_vec(:,iiuav) ) ) );
theta_sigma_bar_w_tilt_2_4 = sigma_bar_w_tilt_squ_2_4(:) .* ( -1 + 2 ./ ( 1 + exp( -alfa_theta_obs_w .* sigma_bar_w_tilt_vec(:,iiuav) ) ) );

== matlab function sim_tase_2025_att_ctrl/cal theta_sigma_bar_w_tilt agent 5 ==
  data: alfa_theta_obs_w input; sigma_bar_w_tilt_squ_1_5 input; theta_sigma_bar_w_tilt_1_5 output; sigma_bar_w_tilt_squ_2_5 input; sigma_bar_w_tilt_vec input; theta_sigma_bar_w_tilt_2_5 output
function [theta_sigma_bar_w_tilt_1_5, theta_sigma_bar_w_tilt_2_5] = fcn(alfa_theta_obs_w, sigma_bar_w_tilt_squ_1_5, sigma_bar_w_tilt_squ_2_5, sigma_bar_w_tilt_vec)
%%%% 计算平滑递增函数
iiuav = 5;
theta_sigma_bar_w_tilt_1_5 = sigma_bar_w_tilt_squ_1_5(:) .* ( -1 + 2 ./ ( 1 + exp( -alfa_theta_obs_w .* sigma_bar_w_tilt_vec(:,iiuav) ) ) );
theta_sigma_bar_w_tilt_2_5 = sigma_bar_w_tilt_squ_2_5(:) .* ( -1 + 2 ./ ( 1 + exp( -alfa_theta_obs_w .* sigma_bar_w_tilt_vec(:,iiuav) ) ) );

== matlab function sim_tase_2025_att_ctrl/choose ksi_est_err 11 ==
  data: x input; y output
function y = fcn(x)
iiuav = 1;
y = x(:,iiuav);

== matlab function sim_tase_2025_att_ctrl/choose ksi_est_err 12 ==
  data: x input; y output
function y = fcn(x)
iiuav = 1;
y = x(:,iiuav);

== matlab function sim_tase_2025_att_ctrl/choose ksi_est_err 13 ==
  data: x input; y output
function y = fcn(x)
iiuav = 2;
y = x(:,iiuav);

== matlab function sim_tase_2025_att_ctrl/choose ksi_est_err 14 ==
  data: x input; y output
function y = fcn(x)
iiuav = 2;
y = x(:,iiuav);

== matlab function sim_tase_2025_att_ctrl/choose ksi_est_err 15 ==
  data: x input; y output
function y = fcn(x)
iiuav = 3;
y = x(:,iiuav);

== matlab function sim_tase_2025_att_ctrl/choose ksi_est_err 16 ==
  data: x input; y output
function y = fcn(x)
iiuav = 3;
y = x(:,iiuav);

== matlab function sim_tase_2025_att_ctrl/choose ksi_est_err 17 ==
  data: x input; y output
function y = fcn(x)
iiuav = 4;
y = x(:,iiuav);

== matlab function sim_tase_2025_att_ctrl/choose ksi_est_err 18 ==
  data: x input; y output
function y = fcn(x)
iiuav = 4;
y = x(:,iiuav);

== matlab function sim_tase_2025_att_ctrl/cal k_1_ij_hat agent 2 ==
  data: k_1_ij_lower input; k_1_ij_hat_node_2 output; k_1_ij_vec input
function k_1_ij_hat_node_2 = fcn(k_1_ij_lower, k_1_ij_vec)
%%%% 计算障碍函数
iiuav = 2;
k_1_ij_hat_node_2 = zeros(3,1);
for jj = 1:3
    k_1_ij_hat_node_2(jj) = (1/2) * ( k_1_ij_vec(jj,iiuav) + k_1_ij_lower(jj,iiuav) );
end

== matlab function sim_tase_2025_att_ctrl/choose ksi_est_err 19 ==
  data: x input; y output
function y = fcn(x)
iiuav = 5;
y = x(:,iiuav);

== matlab function sim_tase_2025_att_ctrl/choose ksi_est_err 20 ==
  data: x input; y output
function y = fcn(x)
iiuav = 5;
y = x(:,iiuav);

== matlab function sim_tase_2025_att_ctrl/combine d_sigma_bar_v_est ==
  data: d_sigma_bar_w_est_1 input; d_sigma_bar_w_est_2 input; d_sigma_bar_w_est_3 input; d_sigma_bar_w_est_4 input; d_sigma_bar_w_est_5 input; d_sigma_bar_w_vec output
function d_sigma_bar_w_vec  = fcn(d_sigma_bar_w_est_1, d_sigma_bar_w_est_2, d_sigma_bar_w_est_3, d_sigma_bar_w_est_4, d_sigma_bar_w_est_5)
%%%% 合并用微分器求得的虚拟速度控制量导数
d_sigma_bar_w_vec = [d_sigma_bar_w_est_1(:), d_sigma_bar_w_est_2(:), d_sigma_bar_w_est_3(:), d_sigma_bar_w_est_4(:), d_sigma_bar_w_est_5(:)];

== matlab function sim_tase_2025_att_ctrl/combine dw_hat ==
  data: dw_hat_1 input; dw_hat_2 input; dw_hat_3 input; dw_hat_4 input; dw_hat_5 input; dw_hat_vec output
function dw_hat_vec  = fcn(dw_hat_1, dw_hat_2, dw_hat_3, dw_hat_4, dw_hat_5)
%%%% 合并扰动观测值dw_hat
dw_hat_vec = [dw_hat_1(:), dw_hat_2(:), dw_hat_3(:), dw_hat_4(:), dw_hat_5(:)];

== matlab function sim_tase_2025_att_ctrl/combine sigma_bar_w_hat ==
  data: sigma_bar_w_hat_1 input; sigma_bar_w_hat_2 input; sigma_bar_w_hat_3 input; sigma_bar_w_hat_4 input; sigma_bar_w_hat_5 input; sigma_bar_w_hat_vec output
function sigma_bar_w_hat_vec  = fcn(sigma_bar_w_hat_1, sigma_bar_w_hat_2, sigma_bar_w_hat_3, sigma_bar_w_hat_4, sigma_bar_w_hat_5)
%%%% 合并虚拟速度控制量观测值sigma_bar_w_hat
sigma_bar_w_hat_vec = [sigma_bar_w_hat_1(:), sigma_bar_w_hat_2(:), sigma_bar_w_hat_3(:), sigma_bar_w_hat_4(:), sigma_bar_w_hat_5(:)];

== matlab function sim_tase_2025_att_ctrl/combine sigma_w ==
  data: sigma_w_1 input; sigma_w_vec output; sigma_w_2 input; sigma_w_3 input; sigma_w_4 input; sigma_w_5 input
function sigma_w_vec = fcn(sigma_w_1, sigma_w_2, sigma_w_3, sigma_w_4, sigma_w_5)
%%%% 合并辅助姿态角速率
sigma_w_vec = [sigma_w_1(:), sigma_w_2(:), sigma_w_3(:), sigma_w_4(:), sigma_w_5(:)];

== matlab function sim_tase_2025_att_ctrl/combine theta_sigma_bar_w_tilt ==
  data: theta_sigma_bar_w_tilt_1_1 input; theta_sigma_bar_w_tilt_1_2 input; theta_sigma_bar_w_tilt_1_3 input; theta_sigma_bar_w_tilt_1_4 input; theta_sigma_bar_w_tilt_1_5 input; theta_sigma_bar_w_tilt_1_vec output; theta_sigma_bar_w_tilt_2_1 input; theta_sigma_bar_w_tilt_2_vec output; theta_sigma_bar_w_tilt_2_2 input; theta_sigma_bar_w_tilt_2_3 input; theta_sigma_bar_w_tilt_2_4 input; theta_sigma_bar_w_tilt_2_5 input
function [theta_sigma_bar_w_tilt_1_vec, theta_sigma_bar_w_tilt_2_vec]  = fcn(theta_sigma_bar_w_tilt_1_1, theta_sigma_bar_w_tilt_1_2, theta_sigma_bar_w_tilt_1_3, theta_sigma_bar_w_tilt_1_4, theta_sigma_bar_w_tilt_1_5, ...
                                                                                                                                            theta_sigma_bar_w_tilt_2_1, theta_sigma_bar_w_tilt_2_2, theta_sigma_bar_w_tilt_2_3, theta_sigma_bar_w_tilt_2_4, theta_sigma_bar_w_tilt_2_5)
%%%% 合并领导者位置观测器输出结果
theta_sigma_bar_w_tilt_1_vec = [theta_sigma_bar_w_tilt_1_1(:), theta_sigma_bar_w_tilt_1_2(:), theta_sigma_bar_w_tilt_1_3(:), theta_sigma_bar_w_tilt_1_4(:), theta_sigma_bar_w_tilt_1_5(:)];
theta_sigma_bar_w_tilt_2_vec = [theta_sigma_bar_w_tilt_2_1(:), theta_sigma_bar_w_tilt_2_2(:), theta_sigma_bar_w_tilt_2_3(:), theta_sigma_bar_w_tilt_2_4(:), theta_sigma_bar_w_tilt_2_5(:)];

== matlab function sim_tase_2025_att_ctrl/trans to column51 ==
  data: x input; y output
function y = fcn(x)
y = x(:);

== matlab function sim_tase_2025_att_ctrl/cal k_1_ij_hat agent 3 ==
  data: k_1_ij_lower input; k_1_ij_hat_node_3 output; k_1_ij_vec input
function k_1_ij_hat_node_3 = fcn(k_1_ij_lower, k_1_ij_vec)
%%%% 计算障碍函数
iiuav = 3;
k_1_ij_hat_node_3 = zeros(3,1);
for jj = 1:3
    k_1_ij_hat_node_3(jj) = (1/2) * ( k_1_ij_vec(jj,iiuav) + k_1_ij_lower(jj,iiuav) );
end

== matlab function sim_tase_2025_att_ctrl/trans to column52 ==
  data: x input; y output
function y = fcn(x)
y = x(:);

== matlab function sim_tase_2025_att_ctrl/trans to column53 ==
  data: x input; y output
function y = fcn(x)
y = x(:);

== matlab function sim_tase_2025_att_ctrl/trans to column54 ==
  data: x input; y output
function y = fcn(x)
y = x(:);

== matlab function sim_tase_2025_att_ctrl/trans to column55 ==
  data: x input; y output
function y = fcn(x)
y = x(:);

== matlab function sim_tase_2025_att_ctrl/trans to column56 ==
  data: x input; y output
function y = fcn(x)
y = x(:);

== matlab function sim_tase_2025_att_ctrl/trans to column57 ==
  data: x input; y output
function y = fcn(x)
y = x(:);

== matlab function sim_tase_2025_att_ctrl/trans to column58 ==
  data: x input; y output
function y = fcn(x)
y = x(:);

== matlab function sim_tase_2025_att_ctrl/trans to column59 ==
  data: x input; y output
function y = fcn(x)
y = x(:);

== matlab function sim_tase_2025_att_ctrl/trans to column60 ==
  data: x input; y output
function y = fcn(x)
y = x(:);

== matlab function sim_tase_2025_att_ctrl/depart k_1_ij 4 ==
  data: y output; x input
function y = fcn(x)
y = x(:,4);

end

== matlab function sim_tase_2025_att_ctrl/depart k_1_ij_hat 5 ==
  data: y output; x input
function y = fcn(x)
y = x(:,5);

end

== matlab function sim_tase_2025_att_ctrl/cal k_1_ij_hat agent 4 ==
  data: k_1_ij_lower input; k_1_ij_hat_node_4 output; k_1_ij_vec input
function k_1_ij_hat_node_4 = fcn(k_1_ij_lower, k_1_ij_vec)
%%%% 计算障碍函数
iiuav = 4;
k_1_ij_hat_node_4 = zeros(3,1);
for jj = 1:3
    k_1_ij_hat_node_4(jj) = (1/2) * ( k_1_ij_vec(jj,iiuav) + k_1_ij_lower(jj,iiuav) );
end

== matlab function sim_tase_2025_att_ctrl/depart k_1_ij_hat 1 ==
  data: y output; x input
function y = fcn(x)
y = x(:,1);

end

== matlab function sim_tase_2025_att_ctrl/depart k_1_ij_hat 2 ==
  data: y output; x input
function y = fcn(x)
y = x(:,2);

end

== matlab function sim_tase_2025_att_ctrl/depart k_1_ij_hat 3 ==
  data: y output; x input
function y = fcn(x)
y = x(:,3);

end

== matlab function sim_tase_2025_att_ctrl/depart k_1_ij_hat 4 ==
  data: y output; x input
function y = fcn(x)
y = x(:,4);

end

== matlab function sim_tase_2025_att_ctrl/depart q_ij_hat 5 ==
  data: y output; x input
function y = fcn(x)
y = x(:,5);

end

== matlab function sim_tase_2025_att_ctrl/depart q_ij_hat 1 ==
  data: y output; x input
function y = fcn(x)
y = x(:,1);

end

== matlab function sim_tase_2025_att_ctrl/depart q_ij_hat 2 ==
  data: y output; x input
function y = fcn(x)
y = x(:,2);

end

== matlab function sim_tase_2025_att_ctrl/depart q_ij_hat 3 ==
  data: y output; x input
function y = fcn(x)
y = x(:,3);

end

== matlab function sim_tase_2025_att_ctrl/depart q_ij_hat 4 ==
  data: y output; x input
function y = fcn(x)
y = x(:,4);

end

== matlab function sim_tase_2025_att_ctrl/combine tau1 ==
  data: dw_1 input; dw_vec output; dw_2 input; dw_3 input; dw_4 input; dw_5 input
function dw_vec = fcn(dw_1, dw_2, dw_3, dw_4, dw_5)
%%%% 合并辅助姿态角速率
dw_vec = [dw_1(:), dw_2(:), dw_3(:), dw_4(:), dw_5(:)];

== matlab function sim_tase_2025_att_ctrl/generate angular rate disturbance agent 1 ==
  data: dw_1 output; dw_aa_t input; dw_ff_t input; dw_phi_t input; t input
function dw_1 = fcn(dw_aa_t, dw_ff_t, dw_phi_t, t)
%%%% 姿态动力学方程中的扰动项设置
epsil_t = zeros(3, 1);

for kk = 1:5
    epsil_t = epsil_t + dw_aa_t(:, kk) .* sin( 2 * pi * dw_ff_t(:, kk) * t + dw_phi_t(:, kk) );
end

dw_1 = [ epsil_t(1) + 1.6 * sin( 0.4 * t ) + 2.0 * cos( 0.5 * t ) + 1.4 * sin( 0.7 * t ) ...
                + 4 * exp( -0.1 * t ) * sin( 0.8 * t ) + 3 / ( 1 + exp( -0.2 * ( t - 15 ) ) ); ...
                epsil_t(2) + 1.2 * sin( 0.2 * t ) + 3 * cos( 0.4 * t ) + 0.8 * sin( 0.6 * t ) ...
                + 2 * exp( -0.15 * t ) * cos( 1.2 * t ) + 3 / ( 1 + exp( -0.3 * ( t - 25 ) ) ); ...
                epsil_t(3) + 1.8 * sin( 0.2 * t ) + 1.6 * sin( 0.3 * t ) + 1.6 * cos( 0.4 * t ) ...
                + 4 * exp( -0.05 * t ) * sin( 0.5 * t + pi / 4 ) + 3 / ( 1 + exp( -0.5 * ( t - 20 ) ) ) ];

== matlab function sim_tase_2025_att_ctrl/cal k_1_ij_hat agent 5 ==
  data: k_1_ij_lower input; k_1_ij_hat_node_5 output; k_1_ij_vec input
function k_1_ij_hat_node_5 = fcn(k_1_ij_lower, k_1_ij_vec)
%%%% 计算障碍函数
iiuav = 5;
k_1_ij_hat_node_5 = zeros(3,1);
for jj = 1:3
    k_1_ij_hat_node_5(jj) = (1/2) * ( k_1_ij_vec(jj,iiuav) + k_1_ij_lower(jj,iiuav) );
end

== matlab function sim_tase_2025_att_ctrl/generate angular rate disturbance agent 2 ==
  data: dw_2 output; dw_aa_t input; dw_ff_t input; dw_phi_t input; t input
function dw_2 = fcn(dw_aa_t, dw_ff_t, dw_phi_t, t)
%%%% 姿态动力学方程中的扰动项设置
epsil_t = zeros(3, 1);

for kk = 1:5
    epsil_t = epsil_t + dw_aa_t(:, kk) .* sin( 2 * pi * dw_ff_t(:, kk) * t + dw_phi_t(:, kk) );
end

dw_2 = [ epsil_t(1) + 1.6 * sin( 0.2 * t ) + 2.0 * cos( 0.3 * t ) + 1.4 * sin( 0.5 * t ) ...
                + 4 * exp( -0.1 * t ) * sin( 0.5 * t ) + 3 / ( 1 + exp( -0.2 * ( t - 15 ) ) ); ...
                epsil_t(2) + 1.2 * sin( 0.1 * t ) + 3 * cos( 0.2 * t ) + 0.8 * sin( 0.4 * t ) ...
                + 2 * exp( -0.15 * t ) * cos( 0.6 * t ) + 3 / ( 1 + exp( -0.3 * ( t - 25 ) ) ); ...
                epsil_t(3) + 1.8 * sin( 0.1 * t ) + 1.6 * sin( 0.2 * t ) + 1.6 * cos( 0.3 * t ) ...
                + 4 * exp( -0.05 * t ) * sin( 0.4 * t + pi / 4 ) + 3 / ( 1 + exp( -0.5 * ( t - 20 ) ) ) ];
